simulink model "Payload_Simulation_Batch"  (R2023b)
settings: Solver=ode15s  StartTime=0.0  StopTime=200  RelTol=1e-3
values from neighbouring files (symbols this model uses):
  ADrogueSide = ADrogueTop / 2    (= 0.0570048194175)    [Payload_BatchSim.m]
  ADrogueTop = pi * (drogueDiameter / (2 * 39.37)) ^ 2    (= 0.114009638835)    [Payload_BatchSim.m]
  AMainSideFinal = AMainTopFinal / 2    (= 3.64830844272)    [Payload_BatchSim.m]
  AMainSideInitial = (mainPackingLength / 39.37) * (innerDiameter / 39.37)    (= 0.0419355677421)    [Payload_BatchSim.m]
  AMainTopFinal = pi * (mainDiameter / (2 * 39.37)) ^ 2    (= 7.29661688544)    [Payload_BatchSim.m]
  AMainTopInitial = pi * (innerDiameter / (2 * 39.37)) ^ 2    (= 0.0126677376483)    [Payload_BatchSim.m]
  ASide = (averageLength / 39.37) * (outerDiameter / 39.37)    (= 0.289065094259)    [Payload_BatchSim.m]
  ATop = pi * (outerDiameter / (2 * 39.37)) ^ 2    (= 0.0134392028711)    [Payload_BatchSim.m]
  CdDrogueSideValue = 1.2    [Payload_BatchSim.m]
  CdDrogueTopValue = 2.65    [Payload_BatchSim.m]
  CdMainSideValue = 0.8    [Payload_BatchSim.m]
  CdMainTopValue = 1.5    [Payload_BatchSim.m]
  CdSide = 0.750    (= 0.75)    [Payload_BatchSim.m]
  CdTop = 0.5    [Payload_BatchSim.m]
  mainDeployFullyAltitude = 600 / 3.281    (= 182.871075891)    [Payload_BatchSim.m]
  mainDeployInitialAltitude = 700 / 3.281    (= 213.34958854)    [Payload_BatchSim.m]
  payloadMass = 0 / 2.205    (= 0)    [Payload_BatchSim.m]
  payloadReleaseAlt = 400 / 3.281    (= 121.914050594)    [Payload_BatchSim.m]
  payloadWeight = payloadMass * g    (= 0)    [Payload_BatchSim.m]
  thetaInitial = angles(i)    [Payload_BatchSim.m]
  windSpeed = windspeeds(i)    [Payload_BatchSim.m]
settings Model: PacingRate=0.890000  Creator=user  LastModifiedBy=Ryan F
settings SolverCC: AlgebraicLoopSolver=TrustRegion
settings DebuggingCC: UnconnectedInputMsg=warning  UnconnectedOutputMsg=warning  UnconnectedLineMsg=warning
settings ModelReferenceCC: EnableRefExpFcnMdlSchedulingChecks=on
settings RTWCC: DLArmComputeVersion=19.05

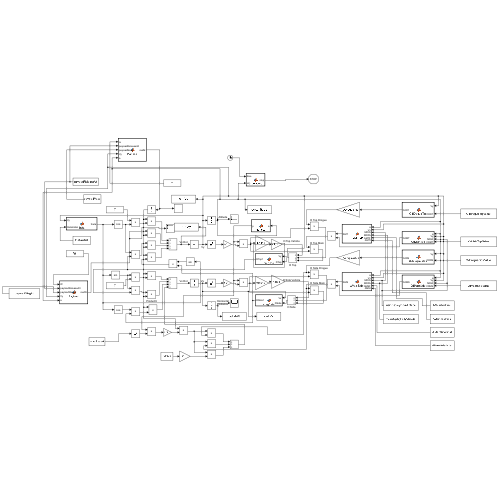
[thumbnail: Simulink's stored preview of the top-level diagram]
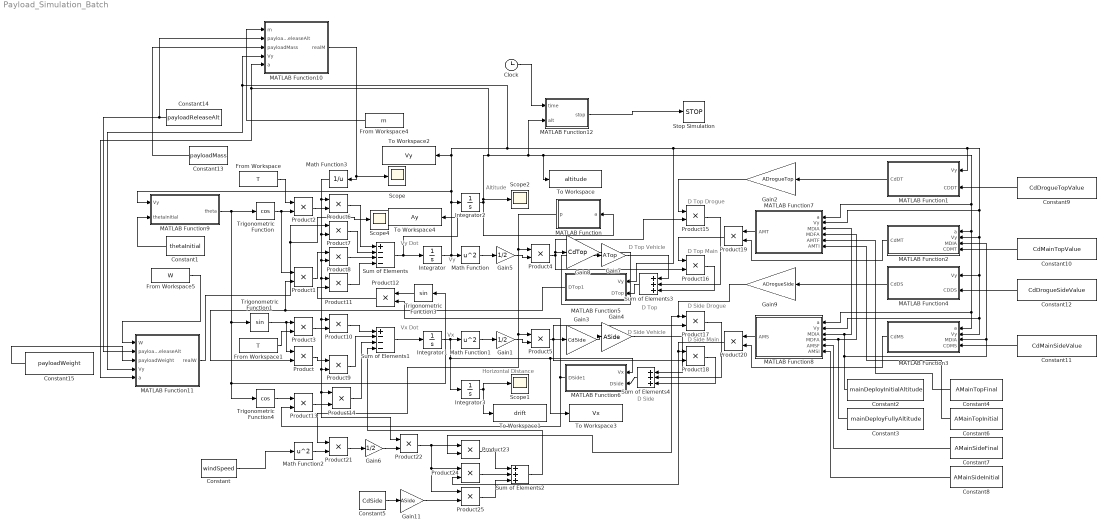
== system Payload_Simulation_Batch ==
  note: D Top Vehicle
  note: Vy Dot
  note: Vx Dot
  note: Vy
  note: Vx
  note: Altitude
  note: Horizontal
      | Distance
  note: D Side Vehicle
  note: D Top Drogue
  note: D Top Main
  note: D Top
  note: D Side Drogue
  note: D Side Main
  note: D Side
  Clock : Clock
  Constant : Constant  Value=windSpeed
  Constant1 : Constant  Value=thetaInitial
  Constant10 : Constant  Value=CdMainTopValue
  Constant11 : Constant  Value=CdMainSideValue
  Constant12 : Constant  Value=CdDrogueSideValue
  Constant13 : Constant  Value=payloadMass
  Constant14 : Constant  Value=payloadReleaseAlt
  Constant15 : Constant  Value=payloadWeight
  Constant2 : Constant  Value=mainDeployInitialAltitude
  Constant3 : Constant  Value=mainDeployFullyAltitude
  Constant4 : Constant  Value=AMainTopFinal
  Constant5 : Constant  Value=CdSide
  Constant6 : Constant  Value=AMainTopInitial
  Constant7 : Constant  Value=AMainSideFinal
  Constant8 : Constant  Value=AMainSideInitial
  Constant9 : Constant  Value=CdDrogueTopValue
  From Workspace : FromWorkspace  VariableName=T  OutputAfterFinalValue=Holding final value
  From Workspace1 : FromWorkspace  VariableName=T  OutputAfterFinalValue=Holding final value
  From Workspace4 : FromWorkspace  VariableName=m  OutputAfterFinalValue=Holding final value
  From Workspace5 : FromWorkspace  VariableName=W  OutputAfterFinalValue=Holding final value
  Gain1 : Gain  Gain=1/2
  Gain11 : Gain  Gain=ASide
  Gain2 : Gain  Gain=ADrogueTop
  Gain3 : Gain  Gain=CdSide
  Gain4 : Gain  Gain=ASide
  Gain5 : Gain  Gain=1/2
  Gain6 : Gain  Gain=1/2
  Gain7 : Gain  Gain=ATop
  Gain8 : Gain  Gain=CdTop
  Gain9 : Gain  Gain=ADrogueSide
  Integrator{,1..3} (4 alike) : Integrator
  MATLAB Function : MATLAB Function  TreatAsAtomicUnit=on
  MATLAB Function1 : MATLAB Function  TreatAsAtomicUnit=on
  MATLAB Function10 : MATLAB Function  TreatAsAtomicUnit=on
  MATLAB Function11 : MATLAB Function  TreatAsAtomicUnit=on
  MATLAB Function12 : MATLAB Function  TreatAsAtomicUnit=on
  MATLAB Function2 : MATLAB Function  TreatAsAtomicUnit=on
  MATLAB Function3 : MATLAB Function  TreatAsAtomicUnit=on
  MATLAB Function4 : MATLAB Function  TreatAsAtomicUnit=on
  MATLAB Function5 : MATLAB Function  TreatAsAtomicUnit=on
  MATLAB Function6 : MATLAB Function  TreatAsAtomicUnit=on
  MATLAB Function7 : MATLAB Function  TreatAsAtomicUnit=on
  MATLAB Function8 : MATLAB Function  TreatAsAtomicUnit=on
  MATLAB Function9 : MATLAB Function  TreatAsAtomicUnit=on
  Math Function : Math  Operator=square
  Math Function1 : Math  Operator=square
  Math Function2 : Math  Operator=square
  Math Function3 : Math  Operator=reciprocal
  Product{,1..25} (26 alike) : Product
  Scope{,1..2,4} (4 alike) : Scope
  Stop Simulation : Stop
  Sum of Elements : Sum  Inputs=+---
  Sum of Elements1 : Sum  Inputs=+---
  Sum of Elements2 : Sum  Inputs=+++
  Sum of Elements3 : Sum  Inputs=+++
  Sum of Elements4 : Sum  Inputs=+++
  To Workspace : ToWorkspace  VariableName=altitude  SampleTime=-1
  To Workspace1 : ToWorkspace  VariableName=drift  SampleTime=-1
  To Workspace2 : ToWorkspace  VariableName=Vy  SampleTime=-1
  To Workspace3 : ToWorkspace  VariableName=Vx  SampleTime=-1
  To Workspace4 : ToWorkspace  VariableName=Ay  SampleTime=-1
  Trigonometric Function : Trigonometry  Operator=cos
  Trigonometric Function1 : Trigonometry
  Trigonometric Function3 : Trigonometry
  Trigonometric Function4 : Trigonometry  Operator=cos
  wires:
  Sum of Elements/1 -> To Workspace4/1, Integrator/1
  Trigonometric Function/1 -> Product2/2, Product1/1
  Product2/1 -> Product6/2
  Product6/1 -> Sum of Elements/1
  Sum of Elements1/1 -> Integrator1/1
  Integrator/1 -> MATLAB Function3/2(Vy), MATLAB Function8/2(Vy), MATLAB Function4/1(Vy), MATLAB Function2/2(Vy), MATLAB Function7/2(Vy), MATLAB Function1/1(Vy), MATLAB Function5/1(Vy), MATLAB Function11/4(Vy), MATLAB Function10/4(Vy), To Workspace2/1, MATLAB Function9/1(Vy), Integrator2/1, Math Function/1
  Trigonometric Function1/1 -> Product3/1, Product/1
  Gain8/1 -> Gain7/1
  Product8/1 -> Sum of Elements/3
  Integrator3/1 -> To Workspace1/1, Scope1/1
  From Workspace/1 -> Product2/1
  From Workspace1/1 -> Product3/2
  From Workspace4/1 -> MATLAB Function10/1(m)
  Math Function3/1 -> Product11/1, Product10/1, Product22/1, Product14/1, Product9/2, Product8/2, Product7/2, Product6/1
  Product7/1 -> Sum of Elements/2
  Product10/1 -> Sum of Elements1/1
  Product9/1 -> Sum of Elements1/2
  Product3/1 -> Product10/2
  Math Function/1 -> Gain5/1
  Math Function1/1 -> Gain1/1
  Product5/1 -> Product17/2, Gain3/1, Product18/2
  Gain3/1 -> Gain4/1
  Product11/1 -> Sum of Elements/4
  MATLAB Function9/1(theta) -> Trigonometric Function4/1, Trigonometric Function3/1, Trigonometric Function1/1, Trigonometric Function/1
  Trigonometric Function3/1 -> Product12/1
  Trigonometric Function4/1 -> Product13/1
  Product14/1 -> Sum of Elements1/3
  Gain5/1 -> Product4/2
  MATLAB Function/1(p) -> Product21/1, Product5/1, Product4/1
  Product4/1 -> Product15/2, Gain8/1, Product16/2
  Gain1/1 -> Product5/2
  Gain2/1 -> Product15/1
  Gain9/1 -> Product23/2, Product17/1
  MATLAB Function4/1(CdDS) -> Gain9/1
  MATLAB Function1/1(CdDT) -> Gain2/1
  Integrator2/1 -> MATLAB Function12/2(alt), MATLAB Function8/1(a), MATLAB Function3/1(a), MATLAB Function2/1(a), MATLAB Function7/1(a), To Workspace/1, MATLAB Function11/5(a), MATLAB Function10/5(a), Scope2/1, MATLAB Function/1(a)
  MATLAB Function5/1(DTop1) -> Product/2, Product1/2
  MATLAB Function6/1(DSide1) -> Product12/2, Product13/2
  Product19/1 -> Product16/1
  Product20/1 -> Product24/2, Product18/1
  MATLAB Function7/1(AMT) -> Product19/1
  MATLAB Function8/1(AMS) -> Product20/1
  MATLAB Function3/1(CdMS) -> Product20/2
  MATLAB Function2/1(CdMT) -> Product19/2
  Integrator1/1 -> Integrator3/1, To Workspace3/1, MATLAB Function6/1(Vx), Math Function1/1
  Constant/1 -> Math Function2/1
  Math Function2/1 -> Product21/2
  Product21/1 -> Gain6/1
  Gain6/1 -> Product22/2
  Product22/1 -> Product25/1, Product24/1, Product23/1
  Constant5/1 -> Gain11/1
  Gain11/1 -> Product25/2
  Product23/1 -> Sum of Elements2/1
  Product24/1 -> Sum of Elements2/2
  Product25/1 -> Sum of Elements2/3
  Sum of Elements2/1 -> Sum of Elements1/4
  Gain7/1 -> Sum of Elements3/1
  Product16/1 -> Sum of Elements3/3
  Product15/1 -> Sum of Elements3/2
  Sum of Elements3/1 -> MATLAB Function5/2(DTop)
  Product1/1 -> Product8/1
  Product12/1 -> Product11/2
  Product13/1 -> Product14/2
  Product/1 -> Product9/1
  Sum of Elements4/1 -> MATLAB Function6/2(DSide)
  Gain4/1 -> Sum of Elements4/1
  Product18/1 -> Sum of Elements4/3
  Product17/1 -> Sum of Elements4/2
  Constant1/1 -> MATLAB Function9/2(thetaInitial)
  Constant2/1 -> MATLAB Function3/3(MDIA), MATLAB Function2/3(MDIA), MATLAB Function8/3(MDIA), MATLAB Function7/3(MDIA)
  Constant3/1 -> MATLAB Function8/4(MDFA), MATLAB Function7/4(MDFA)
  Constant4/1 -> MATLAB Function7/5(AMTF)
  Constant6/1 -> MATLAB Function7/6(AMTI)
  Constant7/1 -> MATLAB Function8/5(AMSF)
  Constant8/1 -> MATLAB Function8/6(AMSI)
  Constant9/1 -> MATLAB Function1/2(CDDT)
  Constant10/1 -> MATLAB Function2/4(CDMT)
  Constant12/1 -> MATLAB Function4/2(CDDS)
  Constant11/1 -> MATLAB Function3/4(CDMS)
  MATLAB Function10/1(realM) -> Scope/1, Math Function3/1
  Constant14/1 -> MATLAB Function11/2(payloadReleaseAlt), MATLAB Function10/2(payloadReleaseAlt)
  Constant13/1 -> MATLAB Function10/3(payloadMass)
  From Workspace5/1 -> MATLAB Function11/1(W)
  Constant15/1 -> MATLAB Function11/3(payloadWeight)
  MATLAB Function11/1(realW) -> Scope4/1, Product7/1
  MATLAB Function12/1(stop) -> Stop Simulation/1
  Clock/1 -> MATLAB Function12/1(time)

== matlab function Payload_Simulation_Batch/MATLAB Function10 ==
  data: m input; payloadReleaseAlt input; realM output; payloadMass input; Vy input; a input
function realM =  Payload( m, payloadReleaseAlt, payloadMass, Vy, a)

if a <= payloadReleaseAlt && Vy < 0   % 
    realM = m - payloadMass;
else
    realM = m;
end

== matlab function Payload_Simulation_Batch/MATLAB Function11 ==
  data: W input; payloadReleaseAlt input; realW output; payloadWeight input; Vy input; a input
function realW =  Payload( W, payloadReleaseAlt, payloadWeight, Vy, a)

if a <= payloadReleaseAlt && Vy < 0
    realW = W - payloadWeight;
    
else
    realW = W;
end

== matlab function Payload_Simulation_Batch/MATLAB Function12 ==
  data: time input; stop output; alt input
function stop = shouldstop(time, alt)
    if time > 10 && alt < 3
        stop = 1;
    else
        stop = 0;
    end

== matlab function Payload_Simulation_Batch/MATLAB Function1 ==
  data: Vy input; CdDT output; CDDT input
function CdDT = CdDrogueTop(Vy, CDDT)
    if Vy < 0 % m/s
        CdDT = CDDT; % unitless
    else
        CdDT = 0; % unitless
    end

== matlab function Payload_Simulation_Batch/MATLAB Function ==
  data: a input; p output
function p = density(a)
    alt = zeros(1, 2001); % m
    temp = zeros(1, 2001); % K
    den = zeros(1, 2001); % kg/m^3
    for i = 0:2000
        alt(i + 1) = round((6371000 / (6371000 + i)) * i);
        temp(i + 1) = ((216.66 - 288.16) / (11000 - 0)) * i + (((288.16 * 11000) - (216.66 * 0)) / (11000 - 0));
        den(i + 1) = (1.2250) * ((temp(alt(i + 1) + 1) / 288.16) .^ -(9.81 / (((temp(alt(i + 1) + 1) - 288.16) / (alt(i + 1) - alt(1))) * 287) + 1));
    end
    den(1) = 1.225;
    p = den(round(a) + 1);

== matlab function Payload_Simulation_Batch/MATLAB Function2 ==
  data: a input; CdMT output; Vy input; MDIA input; CDMT input
function CdMT = CdMainTop(a, Vy, MDIA, CDMT)
    if a <= MDIA && Vy < 0 % m/s
        CdMT = CDMT; % unitless
    else
        CdMT = 0; % unitless
    end

== matlab function Payload_Simulation_Batch/MATLAB Function3 ==
  data: a input; CdMS output; Vy input; MDIA input; CDMS input
function CdMS = CdMainSide(a, Vy, MDIA, CDMS)
    if a <= MDIA && Vy < 0 % m/s
        CdMS = CDMS; % unitless
    else
        CdMS = 0; % unitless
    end

== matlab function Payload_Simulation_Batch/MATLAB Function4 ==
  data: Vy input; CdDS output; CDDS input
function CdDS = CdDrogueSide(Vy, CDDS)
    if Vy < 0 % m/s
        CdDS = CDDS; % unitless
    else
        CdDS = 0; % unitless
    end

== matlab function Payload_Simulation_Batch/MATLAB Function5 ==
  data: Vy input; DTop input; DTop1 output
function DTop1 = dragTop(Vy, DTop)
    if Vy >= 0 % m/s
        DTop1 = DTop; % N
    else
        DTop1 = -DTop; % N
    end

== matlab function Payload_Simulation_Batch/MATLAB Function6 ==
  data: Vx input; DSide input; DSide1 output
function DSide1 = dragSide(Vx, DSide)
    if Vx >= 0 % m/s
        DSide1 = DSide; % N
    else
        DSide1 = -DSide; % N
    end

== matlab function Payload_Simulation_Batch/MATLAB Function7 ==
  data: a input; AMT output; Vy input; MDIA input; MDFA input; AMTF input; AMTI input
function AMT = AMainTop(a, Vy, MDIA, MDFA, AMTF, AMTI)
    k = (1 / (MDFA - MDIA)) * log(AMTF / AMTI);
    C = AMTI * exp(-k * MDIA);
    if a <= MDIA && a >= MDFA && Vy < 0 % m/s
        AMT = C * exp(k * a); % m^2
    elseif a < MDFA && Vy < 0 % m/s
        AMT = AMTF; % m^2
    else
        AMT = AMTI; % m^2
    end

== matlab function Payload_Simulation_Batch/MATLAB Function8 ==
  data: a input; AMS output; Vy input; MDIA input; MDFA input; AMSF input; AMSI input
function AMS = AMainSide(a, Vy, MDIA, MDFA, AMSF, AMSI)
    k = (1 / (MDFA - MDIA)) * log(AMSF / AMSI);
    C = AMSI * exp(-k * MDIA);
    if a <= MDIA && a >= MDFA && Vy < 0 % m/s
        AMS = C * exp(k * a); % m^2
    elseif a < MDFA && Vy < 0 % m/s
        AMS = AMSF; % m^2
    else
        AMS = AMSI; % m^2
    end

== matlab function Payload_Simulation_Batch/MATLAB Function9 ==
  data: Vy input; theta output; thetaInitial input
function theta = theta(Vy, thetaInitial)
    if Vy >= 0 % m/s
        theta = thetaInitial;
    else
        theta = 0;
    end
